simulink model "pidtheetatransform"  (R2014a)
settings: Solver=ode45  StartTime=0.0  StopTime=10.0  RelTol=1e-3
libraries: dspmtrx3 x2
settings Model: Creator=aman  LastModifiedBy=aman

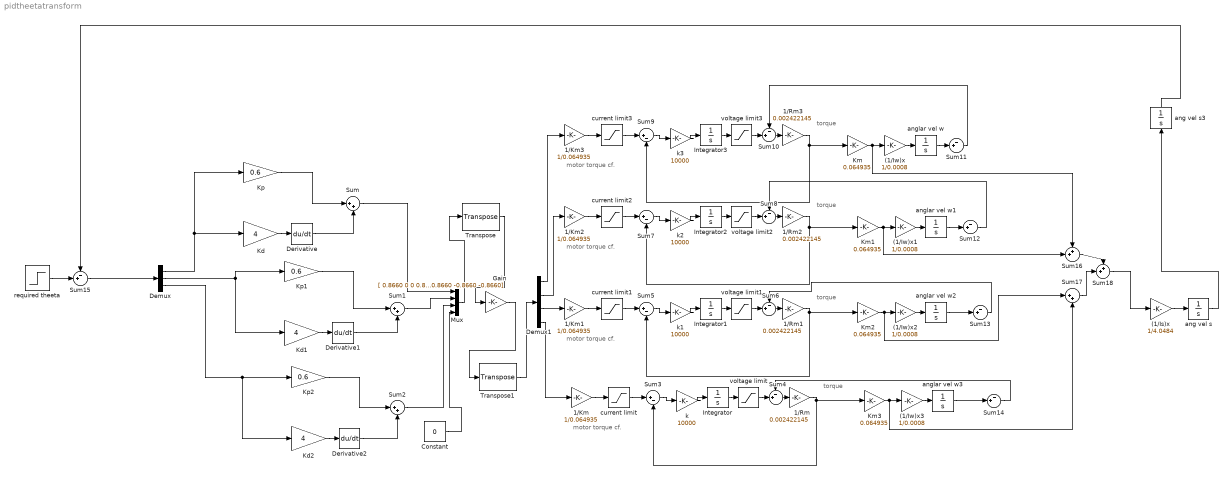
== system pidtheetatransform ==
  note: torque
  note: motor
      | torque
      | cf.
  note: torque
  note: motor
      | torque
      | cf.
  note: torque
  note: motor
      | torque
      | cf.
  note: torque
  note: motor
      | torque
      | cf.
  (1/Is)x : Gain  Gain=1/4.0484
  (1/Iw)x{,1..3} (4 alike) : Gain  Gain=1/0.0008
  1/Km{,1..3} (4 alike) : Gain  Gain=1/0.064935
  1/Rm{,1..3} (4 alike) : Gain  Gain=0.002422145
  Constant : Constant  Value=0
  Demux : Demux  Outputs=3
  Demux1 : Demux
  Derivative : Derivative
  Derivative1 : Derivative
  Derivative2 : Derivative
  Gain : Gain  Gain=|
      | [ 0.8660 0 0 0.8660
      | ; 0.8660 0 0.8660 0 ; 0.86600 0.8660 0 0
      | ;  -0.8660 -0.8660 -0.8660 -0.8660]
  Integrator{,1..3} (4 alike) : Integrator
  Kd : Gain  Gain=4
  Kd1 : Gain  Gain=4
  Kd2 : Gain  Gain=4
  Km{,1..3} (4 alike) : Gain  Gain=0.064935
  Kp : Gain  Gain=0.6
  Kp1 : Gain  Gain=0.6
  Kp2 : Gain  Gain=0.6
  Mux : Mux
  Sum{,1..2,17} (4 alike) : Sum  Inputs=|++
  Sum{4,6,8,10..15} (9 alike) : Sum  Inputs=-+|
  Sum16 : Sum  Inputs=++|
  Sum18 : Sum  Inputs=++|
  Sum{3,5,7,9} (4 alike) : Sum  Inputs=|+-
  Transpose : dspmtrx3/Transpose  Hermitian=off  overflowFlag=off
  Transpose1 : dspmtrx3/Transpose  Hermitian=off  overflowFlag=off
  ang vel s : Integrator
  ang vel s3 : Integrator
  anglar vel w{,1..3} (4 alike) : Integrator
  current limit{,1..3} (4 alike) : Saturate  UpperLimit=0.0816  LowerLimit=-0.016
  k{,1..3} (4 alike) : Gain  Gain=10000
  required theeta : Step  Before=[0 0 0]  After=[0.1 0 0]  SampleTime=0
  voltage limit{,1..3} (4 alike) : Saturate  UpperLimit=34  LowerLimit=-34
  wires:
  Kd/1 -> Derivative/1
  Kp/1 -> Sum/1
  Derivative/1 -> Sum/2
  Demux/1 -> Kp/1, Kd/1
  Kd1/1 -> Derivative1/1
  Kp1/1 -> Sum1/1
  Derivative1/1 -> Sum1/2
  Demux/2 -> Kp1/1, Kd1/1
  Kd2/1 -> Derivative2/1
  Kp2/1 -> Sum2/1
  Derivative2/1 -> Sum2/2
  Demux/3 -> Kd2/1, Kp2/1
  Sum/1 -> Mux/1
  Sum1/1 -> Mux/2
  Sum2/1 -> Mux/3
  1/Km/1 -> current limit/1
  k/1 -> Integrator/1
  Integrator/1 -> voltage limit/1
  1/Rm/1 -> Km3/1, Sum3/2
  current limit/1 -> Sum3/1
  Sum3/1 -> k/1
  Sum4/1 -> 1/Rm/1
  voltage limit/1 -> Sum4/2
  1/Km1/1 -> current limit1/1
  k1/1 -> Integrator1/1
  Integrator1/1 -> voltage limit1/1
  1/Rm1/1 -> Km2/1, Sum5/2
  current limit1/1 -> Sum5/1
  Sum5/1 -> k1/1
  Sum6/1 -> 1/Rm1/1
  voltage limit1/1 -> Sum6/2
  1/Km2/1 -> current limit2/1
  k2/1 -> Integrator2/1
  Integrator2/1 -> voltage limit2/1
  1/Rm2/1 -> Km1/1, Sum7/2
  current limit2/1 -> Sum7/1
  Sum7/1 -> k2/1
  Sum8/1 -> 1/Rm2/1
  voltage limit2/1 -> Sum8/2
  1/Km3/1 -> current limit3/1
  k3/1 -> Integrator3/1
  Integrator3/1 -> voltage limit3/1
  1/Rm3/1 -> Km/1, Sum9/2
  current limit3/1 -> Sum9/1
  Sum9/1 -> k3/1
  Sum10/1 -> 1/Rm3/1
  voltage limit3/1 -> Sum10/2
  Demux1/1 -> 1/Km3/1
  Demux1/2 -> 1/Km2/1
  Demux1/3 -> 1/Km1/1
  Demux1/4 -> 1/Km/1
  anglar vel w/1 -> Sum11/2
  (1/Iw)x/1 -> anglar vel w/1
  Km/1 -> Sum16/1, (1/Iw)x/1
  anglar vel w1/1 -> Sum12/2
  (1/Iw)x1/1 -> anglar vel w1/1
  Km1/1 -> Sum16/2, (1/Iw)x1/1
  anglar vel w2/1 -> Sum13/2
  (1/Iw)x2/1 -> anglar vel w2/1
  Km2/1 -> Sum17/1, (1/Iw)x2/1
  (1/Iw)x3/1 -> anglar vel w3/1
  Km3/1 -> Sum17/2, (1/Iw)x3/1
  anglar vel w3/1 -> Sum14/2
  ang vel s3/1 -> Sum15/1
  required theeta/1 -> Sum15/2
  Sum15/1 -> Demux/1
  Sum11/1 -> Sum10/1
  Sum12/1 -> Sum8/1
  Sum13/1 -> Sum6/1
  Sum14/1 -> Sum4/1
  Sum18/1 -> (1/Is)x/1
  (1/Is)x/1 -> ang vel s/1
  ang vel s/1 -> ang vel s3/1
  Constant/1 -> Mux/4
  Sum16/1 -> Sum18/1
  Sum17/1 -> Sum18/2
  Mux/1 -> Transpose/1
  Transpose/1 -> Gain/1
  Gain/1 -> Transpose1/1
  Transpose1/1 -> Demux1/1
